simulink model "f14_dap"  (Simulink 6.0)
settings: Solver=FixedStepDiscrete  SolverMode=SingleTasking  StartTime=0.0  StopTime=10.0  RelTol=1e-3
PreLoadFcn:
  | f14dat
values from neighbouring files (symbols this model uses):
  deltat = 1    [aero_raddat.m]
  Ka = 0.677    [autopilot_data.mat]    (also in f14dat.m; f14def.m)
  Kf = -1.746    [autopilot_data.mat]    (also in f14dat.m; f14def.m)
  Ki = -3.864    [autopilot_data.mat]    (also in f14dat.m; f14def.m)
  Kq = 0.8156    [autopilot_data.mat]    (also in f14dat.m; f14def.m)
  Tal = 0.3959    [autopilot_data.mat]    (also in f14dat.m; f14def.m)
  Ts = 0.2    [autopilot_data.mat]    (also in f14dat.m = 0.1; f14def.m = 0.1)
  W1 = 2.971    [autopilot_data.mat]    (also in f14dat.m; f14def.m)
  W2 = 4.144    [autopilot_data.mat]    (also in f14dat.m; f14def.m)
undefined symbols (not defined in the file or in its folder): deltat1, DiscIntNeverNeededParam
settings Model: Creator=The MathWorks Inc.  LastModifiedBy=batserve  ExtModeTrigMode=oneshot  ExtModeArmWhenConnect=off  ExtModeAutoUpdateStatusClock=off
settings DataIOCC: LimitDataPoints=off
settings OptimizationCC: BlockReduction=off  BooleanDataType=off
settings DebuggingCC: CheckExecutionContextPreStartOutputMsg=on  CheckExecutionContextRuntimeOutputMsg=on  SolverPrmCheckMsg=none  IntegerOverflowMsg=none
settings HardwareCC: TargetUnknown=on

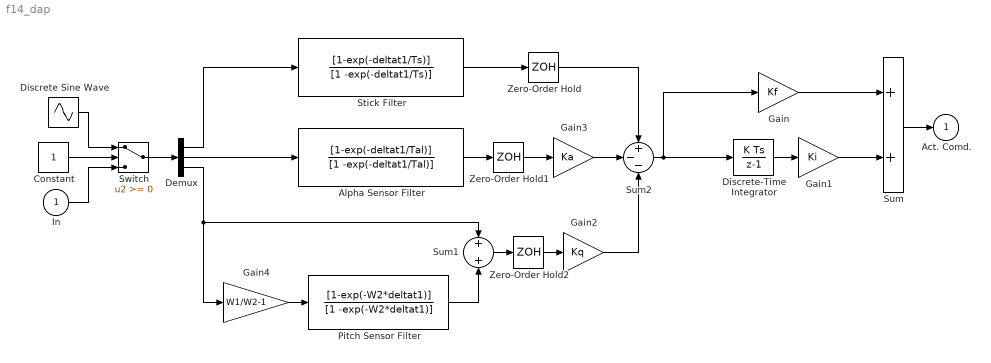
== system f14_dap ==
  In : Inport  Port=1  LatchInput=off
  Alpha Sensor Filter : DiscreteTransferFcn  Numerator=[1-exp(-deltat1/Tal)]  Denominator=[1 -exp(-deltat1/Tal)]  SampleTime=deltat1
  Constant : Constant
  Demux : Demux  Outputs=3
  Discrete Sine Wave : Sin  Frequency=[1 2 3]  SampleTime=deltat1
  Discrete-Time Integrator : DiscreteIntegrator  SampleTime=deltat  ICPrevOutput=DiscIntNeverNeededParam  ICPrevScaledInput=DiscIntNeverNeededParam
  Gain : Gain  Gain=Kf  SaturateOnIntegerOverflow=on
  Gain1 : Gain  Gain=Ki  SaturateOnIntegerOverflow=on
  Gain2 : Gain  Gain=Kq  SaturateOnIntegerOverflow=on
  Gain3 : Gain  Gain=Ka  SaturateOnIntegerOverflow=on
  Gain4 : Gain  Gain=W1/W2-1  SaturateOnIntegerOverflow=on
  Pitch Sensor Filter : DiscreteTransferFcn  Numerator=[1-exp(-W2*deltat1)]  Denominator=[1 -exp(-W2*deltat1)]  SampleTime=deltat1
  Stick Filter : DiscreteTransferFcn  Numerator=[1-exp(-deltat1/Ts)]  Denominator=[1 -exp(-deltat1/Ts)]  SampleTime=deltat1
  Sum : Sum  Inputs=2  SaturateOnIntegerOverflow=on  InputSameDT=on
  Sum1 : Sum  Inputs=2  SaturateOnIntegerOverflow=on  InputSameDT=on
  Sum2 : Sum  Inputs=+--  SaturateOnIntegerOverflow=on  InputSameDT=on
  Switch : Switch  SaturateOnIntegerOverflow=on  InputSameDT=on
  Zero-Order Hold : ZeroOrderHold  SampleTime=deltat
  Zero-Order Hold1 : ZeroOrderHold  SampleTime=deltat
  Zero-Order Hold2 : ZeroOrderHold  SampleTime=deltat
  Act. Comd. : Outport  InitialOutput=0
  wires:
  Gain2/1 -> Sum2/3
  Sum2/1 -> Gain/1, Discrete-Time Integrator/1
  Demux/2 -> Alpha Sensor Filter/1
  Demux/3 -> Sum1/1, Gain4/1
  Demux/1 -> Stick Filter/1
  Stick Filter/1 -> Zero-Order Hold/1
  Zero-Order Hold/1 -> Sum2/1
  Alpha Sensor Filter/1 -> Zero-Order Hold1/1
  Zero-Order Hold1/1 -> Gain3/1
  Sum1/1 -> Zero-Order Hold2/1
  Switch/1 -> Demux/1
  Pitch Sensor Filter/1 -> Sum1/2
  Gain4/1 -> Pitch Sensor Filter/1
  Zero-Order Hold2/1 -> Gain2/1
  Gain3/1 -> Sum2/2
  Sum/1 -> Act. Comd./1
  Discrete-Time Integrator/1 -> Gain1/1
  Gain/1 -> Sum/1
  Gain1/1 -> Sum/2
  In/1 -> Switch/3
  Constant/1 -> Switch/2
  Discrete Sine Wave/1 -> Switch/1
